simulink model "PID_PAL"  (R2015a)
settings: Solver=ode3  StartTime=0.0  StopTime=30  FixedStep=0.1  RelTol=1e-3
libraries: simulink x1
settings Model: Creator=adeca  LastModifiedBy=CARVALHO
settings DataIOCC: SignalLoggingSaveFormat=ModelDataLogs
settings OptimizationCC: ExpressionDepthLimit=2147483647  InitFltsAndDblsToZero=on
settings DebuggingCC: UnderspecifiedInitializationDetection=Classic  MergeDetectMultiDrivingBlocksExec=none  SolverPrmCheckMsg=warning  FcnCallInpInsideContextMsg=UseLocalSettings  StateNameClashWarn=warning
settings GRTTargetCC: CombineOutputUpdateFcns=off  GRTInterface=on

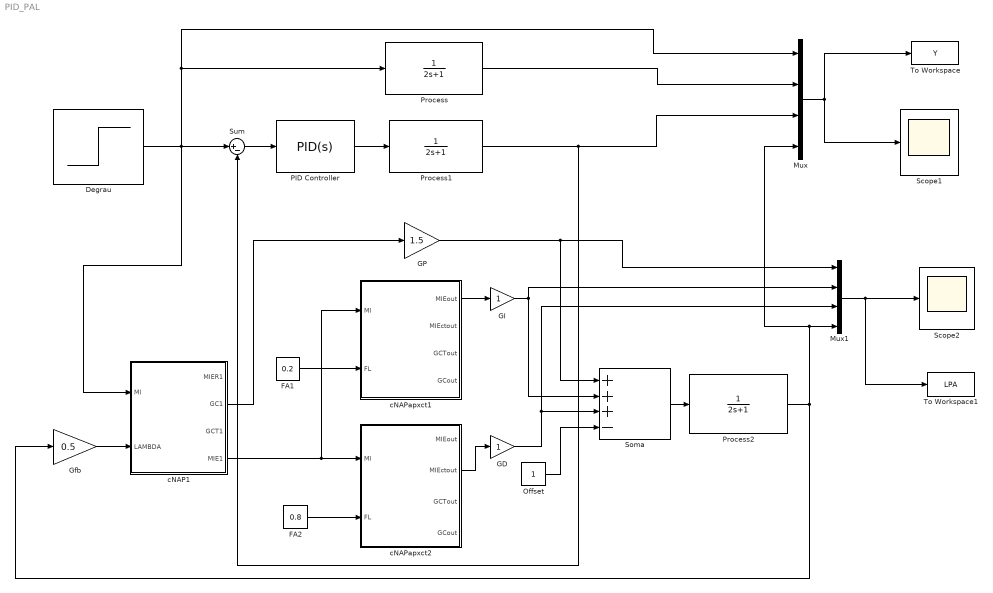
== system PID_PAL ==
  Degrau : Step  Time=15  Before=0.2  After=0.8  SampleTime=0
  FA1 : Constant  Value=0.2
  FA2 : Constant  Value=0.8
  GD : Gain
  GI : Gain
  GP : Gain  Gain=1.5
  Gfb : Gain  Gain=0.5
  Mux : Mux
  Mux1 : Mux
  Offset : Constant
  PID Controller : simulink/Continuous/PID Controller  Controller=PID  TimeDomain=Continuous-time  SampleTime=-1  IntegratorMethod=Forward Euler  FilterMethod=Forward Euler  Form=Parallel  UseFilter=on  ControllerParametersSource=internal  P=1.674  I=1.055  D=0.230  N=1.5  InitialConditionSource=internal  InitialConditionForIntegrator=0  InitialConditionForFilter=0  ExternalReset=none  LimitOutput=off  UpperSaturationLimit=inf  LowerSaturationLimit=-inf  LinearizeAsGain=on  AntiWindupMode=none  Kb=1  TrackingMode=off  Kt=1  PParamMin=[]  PParamMax=[]  IParamMin=[]  IParamMax=[]  DParamMin=[]  DParamMax=[]  NParamMin=[]  NParamMax=[]  KbParamMin=[]  KbParamMax=[]  KtParamMin=[]  KtParamMax=[]  POutMin=[]  POutMax=[]  IOutMin=[]  IOutMax=[]  DOutMin=[]  DOutMax=[]  NOutMin=[]  NOutMax=[]  KbOutMin=[]  KbOutMax=[]  KtOutMin=[]  KtOutMax=[]  IntegratorOutMin=[]  IntegratorOutMax=[]  FilterOutMin=[]  FilterOutMax=[]  SumOutMin=[]  SumOutMax=[]  SumI1OutMin=[]  SumI1OutMax=[]  SumI2OutMin=[]  SumI2OutMax=[]  SumI3OutMin=[]  SumI3OutMax=[]  SumDOutMin=[]  SumDOutMax=[]  SaturationOutMin=[]  SaturationOutMax=[]  IntegratorContinuousStateAttributes=''  IntegratorStateMustResolveToSignalObject=off  IntegratorRTWStateStorageClass=Auto  FilterContinuousStateAttributes=''  FilterStateMustResolveToSignalObject=off  FilterRTWStateStorageClass=Auto  DifferentiatorICPrevScaledInput=0  DifferentiatorOutMin=[]  DifferentiatorOutMax=[]
  Process : TransferFcn  Denominator=[2 1]
  Process1 : TransferFcn  Denominator=[2 1]
  Process2 : TransferFcn  Denominator=[2 1]
  Scope1 : Scope
      settings: TimeRange=49.99  YMin=-0.2  YMax=1.2
  Scope2 : Scope
      settings: TimeRange=49.99  YMin=-0.2  YMax=1.2  SaveName=ScopeData2
  Soma : Sum  Inputs=+++-
  Sum : Sum  Inputs=|+-
  To Workspace : ToWorkspace  VariableName=Y  SampleTime=-1
      settings: Save2DSignal=2-D array (concatenate along first dimension)
  To Workspace1 : ToWorkspace  VariableName=LPA  SampleTime=-1
      settings: Save2DSignal=2-D array (concatenate along first dimension)
  cNAP1 : Subsystem  Tag=NAP  Description=Célula de Aprendizagem NAP
  cNAPapxct1 : Subsystem  Tag=NAP  Description=Célula de Aprendizagem NAP
  cNAPapxct2 : Subsystem  Tag=NAP  Description=Célula de Aprendizagem NAP
  wires:
  PID Controller/1 -> Process1/1
  Degrau/1 -> Mux/1, Process/1, cNAP1/1(MI), Sum/1
  Sum/1 -> PID Controller/1
  Process2/1 -> Gfb/1, Mux/4, Mux1/4
  FA1/1 -> cNAPapxct1/2(FL)
  FA2/1 -> cNAPapxct2/2(FL)
  Process1/1 -> Sum/2, Mux/3
  Mux/1 -> Scope1/1, To Workspace/1
  Process/1 -> Mux/2
  Soma/1 -> Process2/1
  Gfb/1 -> cNAP1/2(LAMBDA)
  cNAP1/2(GC1) -> GP/1
  GD/1 -> Mux1/3, Soma/3
  cNAPapxct1/1(MIEout) -> GI/1
  GI/1 -> Mux1/2, Soma/2
  GP/1 -> Mux1/1, Soma/1
  cNAP1/4(MIE1) -> cNAPapxct1/1(MI), cNAPapxct2/1(MI)
  Mux1/1 -> To Workspace1/1, Scope2/1
  cNAPapxct2/2(MIEctout) -> GD/1
  Offset/1 -> Soma/4

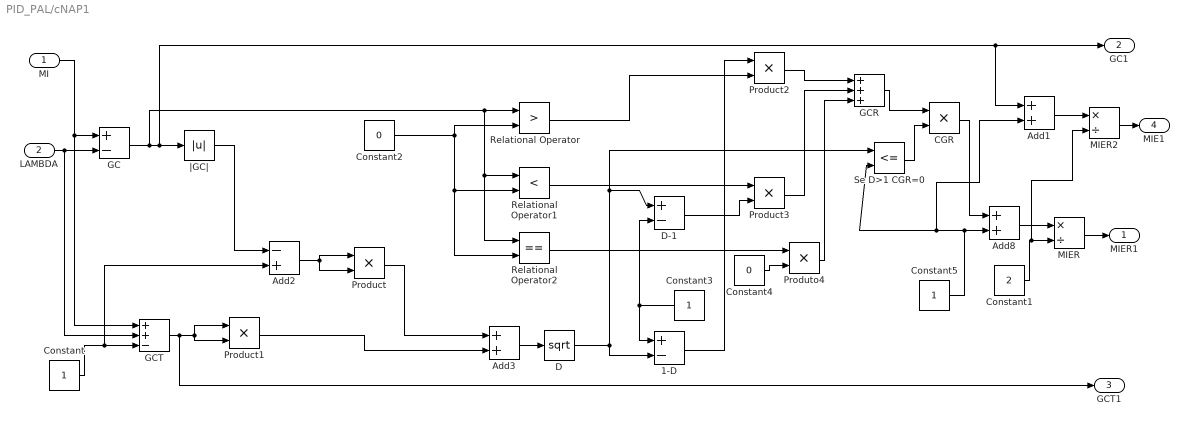
== system PID_PAL/cNAP1 ==
  MI : Inport
  LAMBDA : Inport  Port=2
  1-D : Sum  Inputs=+-
  Add1 : Sum
  Add2 : Sum  Inputs=-+
  Add3 : Sum
  Add8 : Sum
  CGR : Product  RndMeth=Zero
  Constant : Constant
  Constant1 : Constant  Value=2
  Constant2 : Constant  Value=0
  Constant3 : Constant
  Constant4 : Constant  Value=0
  Constant5 : Constant
  D : Math  Operator=sqrt  SaturateOnIntegerOverflow=on
  D-1 : Sum  Inputs=+-
  GC : Sum  Inputs=+-
  GCR : Sum  Inputs=+++
  GCT : Sum  Inputs=++-
  MIER : Product  Inputs=*/
  MIER2 : Product  Inputs=*/
  Product{,1..3} (4 alike) : Product  RndMeth=Zero
  Produto4 : Product  Inputs=**
  Relational Operator : RelationalOperator  Operator=>  OutDataTypeStr=boolean
  Relational Operator1 : RelationalOperator  Operator=<  OutDataTypeStr=boolean
  Relational Operator2 : RelationalOperator  Operator===  OutDataTypeStr=boolean
  Se D>1 CGR=0 : RelationalOperator  Operator=<=  OutDataTypeStr=boolean
  |GC| : Abs
  MIER1 : Outport
  GC1 : Outport  Port=2
  GCT1 : Outport  Port=3
  MIE1 : Outport  Port=4
  wires:
  Constant1/1 -> MIER2/2, MIER/2
  GC/1 -> Relational Operator/1, Relational Operator1/1, Relational Operator2/1, |GC|/1, Add1/1, GC1/1
  Constant/1 -> GCT/3, Add2/2
  |GC|/1 -> Add2/1
  Add2/1 -> Product/1, Product/2
  GCT/1 -> Product1/1, Product1/2, GCT1/1
  Product/1 -> Add3/1
  Product1/1 -> Add3/2
  Constant2/1 -> Relational Operator/2, Relational Operator2/2, Relational Operator1/2
  Relational Operator/1 -> Product2/2
  Constant3/1 -> 1-D/1, D-1/2
  1-D/1 -> Product2/1
  Product2/1 -> GCR/1
  D-1/1 -> Product3/2
  Relational Operator1/1 -> Product3/1
  Product3/1 -> GCR/2
  Constant4/1 -> Produto4/2
  Relational Operator2/1 -> Produto4/1
  Produto4/1 -> GCR/3
  Constant5/1 -> Add8/2, Add1/2, Se D>1 CGR=0/2
  Add8/1 -> MIER/1
  Add3/1 -> D/1
  D/1 -> 1-D/2, D-1/1, Se D>1 CGR=0/1
  MI/1 -> GC/1, GCT/1
  MIER/1 -> MIER1/1
  GCR/1 -> CGR/1
  Se D>1 CGR=0/1 -> CGR/2
  CGR/1 -> Add8/1
  LAMBDA/1 -> GC/2, GCT/2
  Add1/1 -> MIER2/1
  MIER2/1 -> MIE1/1

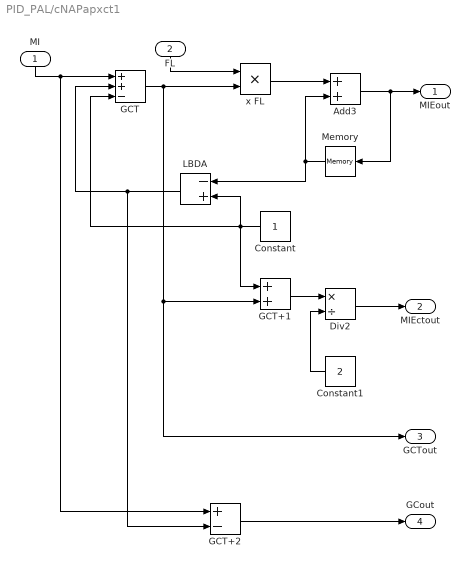
== system PID_PAL/cNAPapxct1 ==
  MI : Inport
  FL : Inport  Port=2
  Add3 : Sum
  Constant : Constant
  Constant1 : Constant  Value=2
  Div2 : Product  Inputs=*/
  GCT : Sum  Inputs=++-
  GCT+1 : Sum
  GCT+2 : Sum  Inputs=+-
  LBDA : Sum  Inputs=-+
  Memory : Memory  X0=0.5  LinearizeAsDelay=on
  x FL : Product  Inputs=**
  MIEout : Outport
  MIEctout : Outport  Port=2
  GCTout : Outport  Port=3
  GCout : Outport  Port=4
  wires:
  MI/1 -> GCT+2/1, GCT/1
  x FL/1 -> Add3/1
  Memory/1 -> Add3/2, LBDA/1
  Add3/1 -> Memory/1, MIEout/1
  LBDA/1 -> GCT+2/2, GCT/2
  Constant/1 -> GCT+1/1, LBDA/2, GCT/3
  GCT/1 -> GCTout/1, GCT+1/2, x FL/2
  FL/1 -> x FL/1
  GCT+1/1 -> Div2/1
  Constant1/1 -> Div2/2
  Div2/1 -> MIEctout/1
  GCT+2/1 -> GCout/1

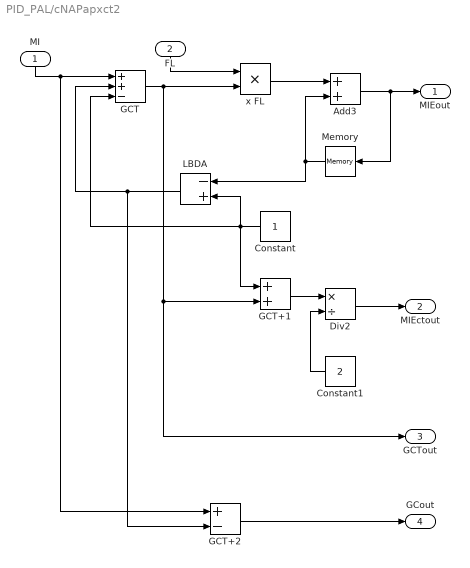
== system PID_PAL/cNAPapxct2 ==
  MI : Inport
  FL : Inport  Port=2
  Add3 : Sum
  Constant : Constant
  Constant1 : Constant  Value=2
  Div2 : Product  Inputs=*/
  GCT : Sum  Inputs=++-
  GCT+1 : Sum
  GCT+2 : Sum  Inputs=+-
  LBDA : Sum  Inputs=-+
  Memory : Memory  X0=0.5  LinearizeAsDelay=on
  x FL : Product  Inputs=**
  MIEout : Outport
  MIEctout : Outport  Port=2
  GCTout : Outport  Port=3
  GCout : Outport  Port=4
  wires:
  MI/1 -> GCT+2/1, GCT/1
  x FL/1 -> Add3/1
  Memory/1 -> Add3/2, LBDA/1
  Add3/1 -> Memory/1, MIEout/1
  LBDA/1 -> GCT+2/2, GCT/2
  Constant/1 -> GCT+1/1, LBDA/2, GCT/3
  GCT/1 -> GCTout/1, GCT+1/2, x FL/2
  FL/1 -> x FL/1
  GCT+1/1 -> Div2/1
  Constant1/1 -> Div2/2
  Div2/1 -> MIEctout/1
  GCT+2/1 -> GCout/1
